simulink model "apilot3"  (Simulink 10.0)
settings: Solver=ode45  StartTime=0.0  StopTime=45  MaxStep=0.033  RelTol=1e-07  AbsTol=1e-05
undefined symbols (not defined in the file): sfunyst
libraries: aplib x11, fbuttons x3, fdclib10 x1
settings Model: Creator=bhisma  LastModifiedBy=bhisma  ExtModeTrigMode=oneshot  ExtModeArmWhenConnect=off
settings DataIOCC: SignalLoggingSaveFormat=ModelDataLogs  SaveOutput=off  SaveTime=off
settings OptimizationCC: BlockReduction=off  BooleanDataType=off  LifeSpan=auto
settings DebuggingCC: SaveWithParameterizedLinksMsg=none  SignalResolutionControl=TryResolveAllWithWarning  MultiTaskDSMMsg=warning  MultiTaskCondExecSysMsg=none  SFUnexpectedBacktrackingDiag=error  SFNoUnconditionalDefaultTransitionDiag=error  SFExecutionAtInitializationDiag=warning  ArithmeticOperatorsInVariantConditions=error
settings HardwareCC: ProdBitPerPointer=64  ProdBitPerSizeT=64  ProdBitPerPtrDiffT=64  ProdLargestAtomicFloat=Float  ProdIntDivRoundTo=Zero  ProdEndianess=LittleEndian  ProdWordSize=64  ProdHWDeviceType=Intel->x86-64 (Windows64)  TargetUnknown=on
settings SFSimCC: SimUseLocalCustomCode=on  CustomCodeUndefinedFunction=FilterOut
settings RTWCC: TemplateMakefile=grt_vc.tmf  RTWUseLocalCustomCode=on
settings CodeAppCC: StateflowObjectComments=off
settings GRTTargetCC: TargetLangStandard=C99 (ISO)
settings ConfigComp: CovMetricSettings=dwe  CovHtmlReporting=off  CovSaveCumulativeToWorkspaceVar=off  CovSaveSingleToWorkspaceVar=off

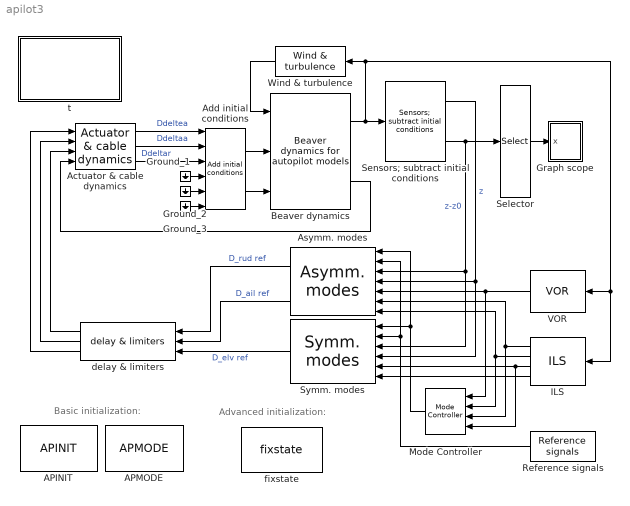
== system apilot3 ==
  note: Basic initialization:
  note: Advanced initialization:
  APINIT : fbuttons/APINIT
  APMODE : fbuttons/APMODE
  Actuator & cable dynamics : aplib/Actuator & cable dynamics
  Add initial conditions : aplib/Add initial conditions
  Asymm. modes : aplib/Asymm. modes
  Beaver dynamics : fdclib10/Beaver dynamics for autopilot models
  Graph scope : Subsystem  mask(Storage scope.){Parameter1=10, Parameter2=-10, Parameter3=10, npts=100, color='g-'}
      mask prompts: Parameter1 "Initial Time Range:"; Parameter2 "Initial y-min:"; Parameter3 "Initial y-max:"; npts "Storage pts.:"; color "Line type (rgbw-.:xo):"
      mask help:
      | Storage scope using MATLAB graph window.
      | Enter plotting ranges and line type.
      mask init:
      | close all; ax = [0, @1, @2, @3];
      mask Help: Uses MATLAB's graph window.\nUse only one block per system.\nLine type must be in quotes.\nSee the M-file sfunyst.m.
      mask Display: plot(0,0,100,100,[83,76,63,52,42,38,28,16,11,84,11,11,11,90,90,11],[75,58,47,54,72,80,84,74,65,65,65,90,40,40,90,90])
  Ground_1 : Ground
  Ground_2 : Ground
  Ground_3 : Ground
  ILS : aplib/ILS
  Mode Controller : aplib/Mode Controller
  Reference signals : aplib/Reference signals
  Selector : Selector  InputPortWidth=13  IndexOptions=Index vector (dialog)  Indices=8  OutputSizes=1
  Sensors; subtract initial conditions : aplib/Sensors; subtract initial conditions
  Symm. modes : aplib/Symm. modes
  VOR : aplib/VOR
  Wind & turbulence : aplib/Wind & turbulence
  delay & limiters : aplib/delay & limiters
  fixstate : fbuttons/fixstate
  t : Subsystem
      settings: OpenFcn=browse apilot
      mask Display: disp('Apilot3\n(complete model)\nMarc Rauw\nApril 2004')
  wires:
  Ground_3/1 -> Add initial conditions/6
  Ground_2/1 -> Add initial conditions/5
  Ground_1/1 -> Add initial conditions/4
  Beaver dynamics/1 -> ILS/1, VOR/1, Wind & turbulence/1, Sensors; subtract initial conditions/1
  Beaver dynamics/2 -> Actuator & cable dynamics/4
  VOR/1 -> Mode Controller/1, Asymm. modes/5
  Symm. modes/1 -> delay & limiters/3  "D_elv ref"
  delay & limiters/3 -> Actuator & cable dynamics/1
  delay & limiters/2 -> Actuator & cable dynamics/2
  delay & limiters/1 -> Actuator & cable dynamics/3
  Reference signals/1 -> Symm. modes/2, Asymm. modes/2
  Mode Controller/1 -> Symm. modes/1, Asymm. modes/1
  Add initial conditions/1 -> Beaver dynamics/2
  Sensors; subtract initial conditions/1 -> Asymm. modes/4, Symm. modes/4  "z"
  Add initial conditions/2 -> Beaver dynamics/3
  Actuator & cable dynamics/1 -> Add initial conditions/1  "Ddeltea"
  Actuator & cable dynamics/2 -> Add initial conditions/2  "Ddeltaa"
  Actuator & cable dynamics/3 -> Add initial conditions/3  "Ddeltar"
  Asymm. modes/1 -> delay & limiters/1  "D_rud ref"
  Asymm. modes/2 -> delay & limiters/2  "D_ail ref"
  Wind & turbulence/1 -> Beaver dynamics/1
  Sensors; subtract initial conditions/2 -> Symm. modes/3, Asymm. modes/3, Selector/1  "z-z0"
  ILS/1 -> Mode Controller/3, Asymm. modes/6
  Selector/1 -> Graph scope/1(x)
  ILS/4 -> Symm. modes/6
  ILS/2 -> Asymm. modes/7, Mode Controller/2
  ILS/3 -> Symm. modes/5, Mode Controller/4

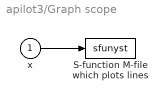
== system apilot3/Graph scope ==
  x : Inport
  "S-function M-file which plots lines " : S-Function  LoadFcn=sfunyst([],[],[],'LoadBlock')  FunctionName=sfunyst  Parameters=ax, color, npts  SFunctionDeploymentMode=off  EnableBusSupport=off
      settings: CopyFcn=sfunyst([],[],[],'CopyBlock')  DeleteFcn=sfunyst([],[],[],'DeleteBlock')
  wires:
  x/1 -> "S-function M-file which plots lines "/1

== system apilot3/t ==
